simulink model "BFE_TestHarness"  (Simulink 8.6)
settings: Solver=FixedStepDiscrete  StartTime=0.0  StopTime=3  FixedStep=Ts  RelTol=1e-3
PreLoadFcn:
  | addpath('MBD_Tests')
  | 
  | load('Workspace\EnvVar.mat')
  | run('MBD_Tests\MBD_tests_init.m')
  | if exist('tl_preloadfcn','file'), tl_preloadfcn(gcs,402); end
PostLoadFcn:
  | if exist('tl_postloadfcn','file'), tl_postloadfcn(gcs,402); end
InitFcn:
  | if exist('tlds_init','file'), tlds_init(gcs); end
StartFcn:
  | if exist('tlds_start','file'), tlds_start(gcs); end
StopFcn:
  | if exist('tlds_stop','file'), tlds_stop(gcs); end
undefined symbols (not defined in the file): ddv, Ts, u2, u3, u4
libraries: tllib x11, simulink x8, LIB_TF_G_111 x2, LIB_TF_G_12_StepControl x2, LIB_TF_G_112 x1, LIB_TF_G_113 x1
(part 11 of 17)

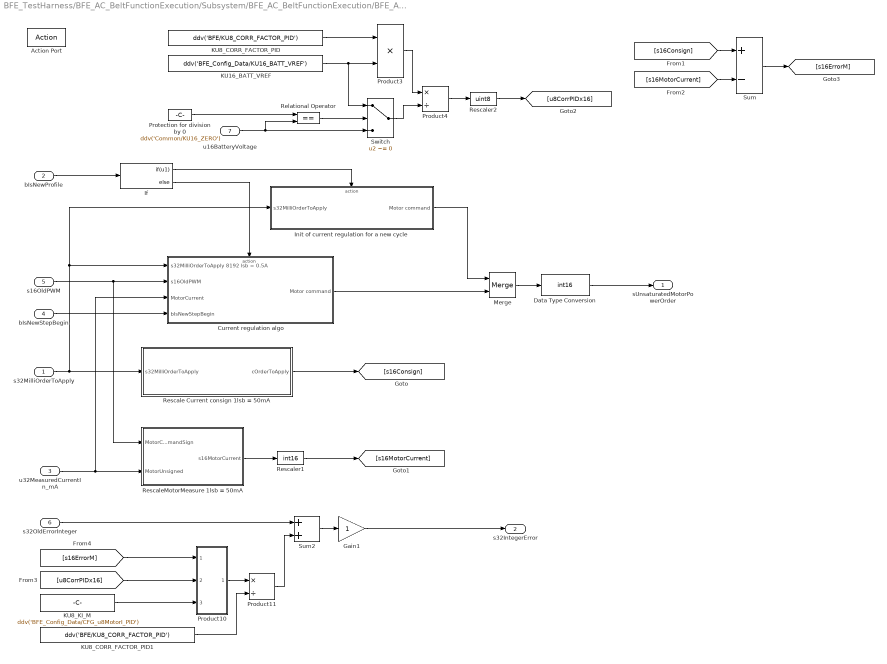
== system BFE_TestHarness/BFE_AC_BeltFunctionExecution/Subsystem/BFE_AC_BeltFunctionExecution/BFE_AC_BeltFunctionExecution/BFE_runExecuteStandardSteps/ExecuteStandardSteps/SubsystemConvertOrderToMotorPower/Current_Regulation/Standard Regulation ==
  s32MilliOrderToApply : Inport  RequirementInfo={} %GIDa_a782df3b_cd2f_48ec_84bc_b42b59744bc6
  bIsNewProfile : Inport  RequirementInfo={} %GIDa_a44577a2_8625_45c3_aeb0_51c9285d1a85  Port=2
  u32MeasuredCurrentIn_mA : Inport  RequirementInfo={} %GIDa_7c33bc16_f4d7_41a6_837e_bf2e5b8e2de6  Port=3
  bIsNewStepBegin : Inport  RequirementInfo={} %GIDa_89b8018c_31ff_454d_820a_6fb8a1af90d7  Port=4
  s16OldPWM : Inport  RequirementInfo={} %GIDa_84405069_397b_4c2d_9940_083b086742df  Port=5
  s32OldErrorInteger : Inport  RequirementInfo={} %GIDa_3b3878a2_30a5_4bd8_a4cc_60f462ef7e39  Port=6
  u16BatteryVoltage : Inport  RequirementInfo={} %GIDa_ae36fff5_70fb_4eda_b8dc_2f0f1fd7ad12  Port=7
  Action Port : ActionPort  RequirementInfo={} %GIDa_eb4ea71c_0e34_4a3e_b607_23ed5579d26c  ActionType=then
  Current regulation algo : Subsystem  TreatAsAtomicUnit=on
  Data Type Conversion : DataTypeConversion  RequirementInfo={} %GIDa_77bacd59_8a03_4be2_81ef_2d2f22f87e72  OutDataTypeStr=int16  mask(TL_Rescaler){data={'date',735951.66854917828}}
      settings: DeleteFcn=if exist('delete_tlblock','file')==2,delete_tlblock(gcbh);end  NameChangeFcn=if exist('rename_tlblock','file')==2,rename_tlblock(gcbh);end  OpenFcn=if exist('tl_open_blockdlg','file')==2,tl_open_blockdlg(gcbh);else,open_system(gcbh,'parameter');end
      mask Help: eval(['if exist(''tl_online_help'',''file'') == 2, tl_online_help(''Topic'',''TL_Rescaler''),else, web([''jar:file:///'',matlabroot,''/help/toolbox/simulink/help.jar!/slref/' lower(get_param(gcbh,'Blocktype')) '.html''], ''-helpbrowser''),end'])
      mask Display: plot([-0.05, 1.05, NaN, -0.05, 1.05],[.01, .01, NaN, .99, .99])
  Gain1 : Gain  RequirementInfo={} %GIDa_240eae8e_68ae_46cb_b8de_0b9900bc89c0  OutDataTypeStr=int32  mask(TL_Gain){data={'output',{'type','Int32'},'date',735951.66854881949}}
      settings: CopyFcn=if exist('tl_reset_reviewflag','file')==2,tl_reset_reviewflag(gcbh);end  DeleteFcn=if exist('delete_tlblock','file')==2,delete_tlblock(gcbh);end  NameChangeFcn=if exist('rename_tlblock','file')==2,rename_tlblock(gcbh);end  OpenFcn=if exist('tl_open_blockdlg','file')==2,tl_open_blockdlg(gcbh);else,open_system(gcbh,'parameter');end
      mask Help: eval(['if exist(''tl_online_help'',''file'') == 2, tl_online_help(''Topic'',''TL_Gain''),else, web([''jar:file:///'',matlabroot,''/help/toolbox/simulink/help.jar!/slref/' lower(get_param(gcbh,'Blocktype')) '.html''], ''-helpbrowser''),end'])
      mask Display: plot([0, .9, 0],[.05, .5, .95])
  If : If  IfExpression=u1
  Init of current regulation for a new cycle : Subsystem  TreatAsAtomicUnit=on
  KU16_BATT_VREF : Constant  RequirementInfo={} %GIDa_2fbae1ab_a28b_4d2e_975d_0f9f269946ee  Value=ddv('BFE_Config_Data/KU16_BATT_VREF')  OutDataTypeStr=uint16  mask(TL_Constant){data={'output',{'variable','BFE_Config_Data/KU16_BATT_VREF'},'date',735951.66854578699}}
      settings: CopyFcn=if exist('tl_reset_reviewflag','file')==2,tl_reset_reviewflag(gcbh);end  DeleteFcn=if exist('delete_tlblock','file')==2,delete_tlblock(gcbh);end  NameChangeFcn=if exist('rename_tlblock','file')==2,rename_tlblock(gcbh);end  OpenFcn=if exist('tl_open_blockdlg','file')==2,tl_open_blockdlg(gcbh);else,open_system(gcbh,'parameter');end
      mask Help: eval(['if exist(''tl_online_help'',''file'') == 2, tl_online_help(''Topic'',''TL_Constant''),else, web([''jar:file:///'',matlabroot,''/help/toolbox/simulink/help.jar!/slref/' lower(get_param(gcbh,'Blocktype')) '.html''], ''-helpbrowser''),end'])
      mask Display: plot([-0.05, 1.05, NaN, -0.05, 1.05],[.01, .01, NaN, .99, .99])
  KU8_CORR_FACTOR_PID : Constant  RequirementInfo={} %GIDa_78255bf5_403f_48d2_a530_3c6e07dfbf1a  Value=ddv('BFE/KU8_CORR_FACTOR_PID')  OutDataTypeStr=uint8  mask(TL_Constant){data={'output',{'variable','BFE/KU8_CORR_FACTOR_PID'},'date',735951.66854541667}}
      settings: CopyFcn=if exist('tl_reset_reviewflag','file')==2,tl_reset_reviewflag(gcbh);end  DeleteFcn=if exist('delete_tlblock','file')==2,delete_tlblock(gcbh);end  NameChangeFcn=if exist('rename_tlblock','file')==2,rename_tlblock(gcbh);end  OpenFcn=if exist('tl_open_blockdlg','file')==2,tl_open_blockdlg(gcbh);else,open_system(gcbh,'parameter');end
      mask Help: eval(['if exist(''tl_online_help'',''file'') == 2, tl_online_help(''Topic'',''TL_Constant''),else, web([''jar:file:///'',matlabroot,''/help/toolbox/simulink/help.jar!/slref/' lower(get_param(gcbh,'Blocktype')) '.html''], ''-helpbrowser''),end'])
      mask Display: plot([-0.05, 1.05, NaN, -0.05, 1.05],[.01, .01, NaN, .99, .99])
  KU8_CORR_FACTOR_PID1 : Constant  RequirementInfo={} %GIDa_3c653f60_82b8_4086_9e8c_c5b737d3d0e8  Value=ddv('BFE/KU8_CORR_FACTOR_PID')  OutDataTypeStr=uint8  mask(TL_Constant){data={'output',{'variable','BFE/KU8_CORR_FACTOR_PID'},'date',735951.66854503471}}
      settings: CopyFcn=if exist('tl_reset_reviewflag','file')==2,tl_reset_reviewflag(gcbh);end  DeleteFcn=if exist('delete_tlblock','file')==2,delete_tlblock(gcbh);end  NameChangeFcn=if exist('rename_tlblock','file')==2,rename_tlblock(gcbh);end  OpenFcn=if exist('tl_open_blockdlg','file')==2,tl_open_blockdlg(gcbh);else,open_system(gcbh,'parameter');end
      mask Help: eval(['if exist(''tl_online_help'',''file'') == 2, tl_online_help(''Topic'',''TL_Constant''),else, web([''jar:file:///'',matlabroot,''/help/toolbox/simulink/help.jar!/slref/' lower(get_param(gcbh,'Blocktype')) '.html''], ''-helpbrowser''),end'])
      mask Display: plot([-0.05, 1.05, NaN, -0.05, 1.05],[.01, .01, NaN, .99, .99])
  KU8_KI_M : Constant  RequirementInfo={} %GIDa_2b7a27a1_c83e_482d_9a98_41e7f4309a04  Value=ddv('BFE_Config_Data/CFG_u8MotorI_PID')  OutDataTypeStr=uint8  mask(TL_Constant){data={'output',{'variable','BFE_Config_Data/CFG_u8MotorI_PID'},'date',735951.66854465276}}
      settings: CopyFcn=if exist('tl_reset_reviewflag','file')==2,tl_reset_reviewflag(gcbh);end  DeleteFcn=if exist('delete_tlblock','file')==2,delete_tlblock(gcbh);end  NameChangeFcn=if exist('rename_tlblock','file')==2,rename_tlblock(gcbh);end  OpenFcn=if exist('tl_open_blockdlg','file')==2,tl_open_blockdlg(gcbh);else,open_system(gcbh,'parameter');end
      mask Help: eval(['if exist(''tl_online_help'',''file'') == 2, tl_online_help(''Topic'',''TL_Constant''),else, web([''jar:file:///'',matlabroot,''/help/toolbox/simulink/help.jar!/slref/' lower(get_param(gcbh,'Blocktype')) '.html''], ''-helpbrowser''),end'])
      mask Display: plot([-0.05, 1.05, NaN, -0.05, 1.05],[.01, .01, NaN, .99, .99])
  Merge : Merge  InitialOutput=0  mask(TL_Merge){data={'date',735951.6685442708}}
      settings: CopyFcn=if exist('tl_reset_reviewflag','file')==2,tl_reset_reviewflag(gcbh);end  DeleteFcn=if exist('delete_tlblock','file')==2,delete_tlblock(gcbh);end  NameChangeFcn=if exist('rename_tlblock','file')==2,rename_tlblock(gcbh);end  OpenFcn=if exist('tl_open_blockdlg','file')==2,tl_open_blockdlg(gcbh);else,open_system(gcbh,'parameter');end
      mask Help: eval(['if exist(''tl_online_help'',''file'') == 2, tl_online_help(''Topic'',''TL_Merge''),else, web([''jar:file:///'',matlabroot,''/help/toolbox/simulink/help.jar!/slref/' lower(get_param(gcbh,'Blocktype')) '.html''], ''-helpbrowser''),end'])
      mask Display: plot([-0.05, 1.05, NaN, -0.05, 1.05],[.01, .01, NaN, .99, .99])
  Product10 : Subsystem  RequirementInfo={} %GIDa_f767c257_68db_48eb_9874_98d302407301
      mask Display: plot([4 10 NaN 4 10 ],[82 88 NaN 88 82 ]);plot([4 10 NaN 4 10 ],[47 53 NaN 53 47 ]);plot([4 10 NaN 4 10 ],[12 18 NaN 18 12 ]);
  Product11 : Product  RequirementInfo={} %GIDa_05da5e16_588f_40e9_b405_55adb34adf78  Inputs=*/  RndMeth=Zero  mask(TL_Product){data={'output',{'type','Int32'},'date',735951.66854312504}}
      settings: CopyFcn=if exist('tl_reset_reviewflag','file')==2,tl_reset_reviewflag(gcbh);end  DeleteFcn=if exist('delete_tlblock','file')==2,delete_tlblock(gcbh);end  NameChangeFcn=if exist('rename_tlblock','file')==2,rename_tlblock(gcbh);end  OpenFcn=if exist('tl_open_blockdlg','file')==2,tl_open_blockdlg(gcbh);else,open_system(gcbh,'parameter');end
      mask Help: eval(['if exist(''tl_online_help'',''file'') == 2, tl_online_help(''Topic'',''TL_Product''),else, web([''jar:file:///'',matlabroot,''/help/toolbox/simulink/help.jar!/slref/' lower(get_param(gcbh,'Blocktype')) '.html''], ''-helpbrowser''),end'])
      mask Display: plot([-0.05, 1.05, NaN, -0.05, 1.05],[.01, .01, NaN, .99, .99])
  Product3 : Product  RequirementInfo={} %GIDa_5e53fb6f_ceab_4fe0_9d47_7ec7af3cf549  Inputs=**  RndMeth=Zero  mask(TL_Product){data={'output',{'type','UInt32'},'date',735951.66854276625}}
      settings: CopyFcn=if exist('tl_reset_reviewflag','file')==2,tl_reset_reviewflag(gcbh);end  DeleteFcn=if exist('delete_tlblock','file')==2,delete_tlblock(gcbh);end  NameChangeFcn=if exist('rename_tlblock','file')==2,rename_tlblock(gcbh);end  OpenFcn=if exist('tl_open_blockdlg','file')==2,tl_open_blockdlg(gcbh);else,open_system(gcbh,'parameter');end
      mask Help: eval(['if exist(''tl_online_help'',''file'') == 2, tl_online_help(''Topic'',''TL_Product''),else, web([''jar:file:///'',matlabroot,''/help/toolbox/simulink/help.jar!/slref/' lower(get_param(gcbh,'Blocktype')) '.html''], ''-helpbrowser''),end'])
      mask Display: plot([-0.05, 1.05, NaN, -0.05, 1.05],[.01, .01, NaN, .99, .99])
  Product4 : Product  RequirementInfo={} %GIDa_70232b70_1706_4488_b9fd_672dede75738  Inputs=*/  RndMeth=Zero  mask(TL_Product){data={'output',{'type','UInt32'},'exceptionhandling',0,'date',735951.66854238429}}
      settings: CopyFcn=if exist('tl_reset_reviewflag','file')==2,tl_reset_reviewflag(gcbh);end  DeleteFcn=if exist('delete_tlblock','file')==2,delete_tlblock(gcbh);end  NameChangeFcn=if exist('rename_tlblock','file')==2,rename_tlblock(gcbh);end  OpenFcn=if exist('tl_open_blockdlg','file')==2,tl_open_blockdlg(gcbh);else,open_system(gcbh,'parameter');end
      mask Help: eval(['if exist(''tl_online_help'',''file'') == 2, tl_online_help(''Topic'',''TL_Product''),else, web([''jar:file:///'',matlabroot,''/help/toolbox/simulink/help.jar!/slref/' lower(get_param(gcbh,'Blocktype')) '.html''], ''-helpbrowser''),end'])
      mask Display: plot([-0.05, 1.05, NaN, -0.05, 1.05],[.01, .01, NaN, .99, .99])
  Protection for division by 0 : Constant  Value=ddv('Common/KU16_ZERO')  mask(TL_Constant){data={'output',{'variable','Common/KU16_ZERO'},'date',735951.66854201385}}
      settings: CopyFcn=if exist('tl_reset_reviewflag','file')==2,tl_reset_reviewflag(gcbh);end  DeleteFcn=if exist('delete_tlblock','file')==2,delete_tlblock(gcbh);end  NameChangeFcn=if exist('rename_tlblock','file')==2,rename_tlblock(gcbh);end  OpenFcn=if exist('tl_open_blockdlg','file')==2,tl_open_blockdlg(gcbh);else,open_system(gcbh,'parameter');end
      mask Help: eval(['if exist(''tl_online_help'',''file'') == 2, tl_online_help(''Topic'',''TL_Constant''),else, web([''jar:file:///'',matlabroot,''/help/toolbox/simulink/help.jar!/slref/' lower(get_param(gcbh,'Blocktype')) '.html''], ''-helpbrowser''),end'])
      mask Display: plot([-0.05, 1.05, NaN, -0.05, 1.05],[.01, .01, NaN, .99, .99])
  Relational Operator : RelationalOperator  Operator===  OutDataTypeStr=boolean  mask(TL_RelationalOperator){data={'date',735951.66854165506}}
      settings: DeleteFcn=if exist('delete_tlblock','file')==2,delete_tlblock(gcbh);end  NameChangeFcn=if exist('rename_tlblock','file')==2,rename_tlblock(gcbh);end  OpenFcn=if exist('tl_open_blockdlg','file')==2,tl_open_blockdlg(gcbh);else,open_system(gcbh,'parameter');end
      mask Help: eval(['if exist(''tl_online_help'',''file'') == 2, tl_online_help(''Topic'',''TL_RelationalOperator''),else, web([''jar:file:///'',matlabroot,''/help/toolbox/simulink/help.jar!/slref/' lower(get_param(gcbh,'Blocktype')) '.html''], ''-helpbrowser''),end'])
      mask Display: plot([-0.05, 1.05, NaN, -0.05, 1.05],[.01, .01, NaN, .99, .99])
  Rescale Current consign 1lsb = 50mA : Subsystem  RequirementInfo={} %GIDa_fdff63d8_bdcf_4376_a137_337af77cbfb4
  RescaleMotorMeasure 1lsb = 50mA : Subsystem  RequirementInfo={} %GIDa_d2c6756e_dc23_445d_b4ca_0746f033342a  TreatAsAtomicUnit=on
  Rescaler1 : DataTypeConversion  RequirementInfo={} %GIDa_044cb36d_c668_4fc2_a10d_86685e254bcb  OutDataTypeStr=int16  SaturateOnIntegerOverflow=on  RndMeth=Zero  mask(TL_Rescaler){data={'output',{'name','s16MotorCurrentM_204'},'date',735951.66853535874}}
      settings: DeleteFcn=if exist('delete_tlblock','file')==2,delete_tlblock(gcbh);end  NameChangeFcn=if exist('rename_tlblock','file')==2,rename_tlblock(gcbh);end  OpenFcn=if exist('tl_open_blockdlg','file')==2,tl_open_blockdlg(gcbh);else,open_system(gcbh,'parameter');end
      mask Help: eval(['if exist(''tl_online_help'',''file'') == 2, tl_online_help(''Topic'',''TL_Rescaler''),else, web([''jar:file:///'',matlabroot,''/help/toolbox/simulink/help.jar!/slref/' lower(get_param(gcbh,'Blocktype')) '.html''], ''-helpbrowser''),end'])
      mask Display: plot([-0.05, 1.05, NaN, -0.05, 1.05],[.01, .01, NaN, .99, .99])
  Rescaler2 : DataTypeConversion  RequirementInfo={} %GIDa_26de5298_a930_4926_bcb3_9f8f9b842192  OutDataTypeStr=uint8  SaturateOnIntegerOverflow=on  RndMeth=Zero  mask(TL_Rescaler){data={'output',{'name','u8CorrPIDx16_204','type','UInt8'},'date',735951.66853504628}}
      settings: DeleteFcn=if exist('delete_tlblock','file')==2,delete_tlblock(gcbh);end  NameChangeFcn=if exist('rename_tlblock','file')==2,rename_tlblock(gcbh);end  OpenFcn=if exist('tl_open_blockdlg','file')==2,tl_open_blockdlg(gcbh);else,open_system(gcbh,'parameter');end
      mask Help: eval(['if exist(''tl_online_help'',''file'') == 2, tl_online_help(''Topic'',''TL_Rescaler''),else, web([''jar:file:///'',matlabroot,''/help/toolbox/simulink/help.jar!/slref/' lower(get_param(gcbh,'Blocktype')) '.html''], ''-helpbrowser''),end'])
      mask Display: plot([-0.05, 1.05, NaN, -0.05, 1.05],[.01, .01, NaN, .99, .99])
  Sum : Sum  RequirementInfo={} %GIDa_21aea4e4_1c5d_4da0_972e_0efc7a1f84ed  Inputs=+-  mask(TL_Sum){data={'output',{'name','s16ErrorM_204'},'date',735951.66853471065}}
      settings: CopyFcn=if exist('tl_reset_reviewflag','file')==2,tl_reset_reviewflag(gcbh);end  DeleteFcn=if exist('delete_tlblock','file')==2,delete_tlblock(gcbh);end  NameChangeFcn=if exist('rename_tlblock','file')==2,rename_tlblock(gcbh);end  OpenFcn=if exist('tl_open_blockdlg','file')==2,tl_open_blockdlg(gcbh);else,open_system(gcbh,'parameter');end
      mask Help: eval(['if exist(''tl_online_help'',''file'') == 2, tl_online_help(''Topic'',''TL_Sum''),else, web([''jar:file:///'',matlabroot,''/help/toolbox/simulink/help.jar!/slref/' lower(get_param(gcbh,'Blocktype')) '.html''], ''-helpbrowser''),end'])
      mask Display: plot([-0.05, 1.05, NaN, -0.05, 1.05],[.01, .01, NaN, .99, .99])
  Sum2 : Sum  RequirementInfo={} %GIDa_070b8bc6_ad2d_4c77_accf_3ff0a1d37eb1  mask(TL_Sum){data={'output',{'type','Int32'},'date',735951.66853435186}}
      settings: CopyFcn=if exist('tl_reset_reviewflag','file')==2,tl_reset_reviewflag(gcbh);end  DeleteFcn=if exist('delete_tlblock','file')==2,delete_tlblock(gcbh);end  NameChangeFcn=if exist('rename_tlblock','file')==2,rename_tlblock(gcbh);end  OpenFcn=if exist('tl_open_blockdlg','file')==2,tl_open_blockdlg(gcbh);else,open_system(gcbh,'parameter');end
      mask Help: eval(['if exist(''tl_online_help'',''file'') == 2, tl_online_help(''Topic'',''TL_Sum''),else, web([''jar:file:///'',matlabroot,''/help/toolbox/simulink/help.jar!/slref/' lower(get_param(gcbh,'Blocktype')) '.html''], ''-helpbrowser''),end'])
      mask Display: plot([-0.05, 1.05, NaN, -0.05, 1.05],[.01, .01, NaN, .99, .99])
  Switch : Switch  Criteria=u2 ~= 0  mask(TL_Switch){data={'output',{'name','u16BattVoltFiltered_$B','type','UInt16'},'date',735951.66853395838}}
      settings: CopyFcn=if exist('tl_reset_reviewflag','file')==2,tl_reset_reviewflag(gcbh);end  DeleteFcn=if exist('delete_tlblock','file')==2,delete_tlblock(gcbh);end  NameChangeFcn=if exist('rename_tlblock','file')==2,rename_tlblock(gcbh);end  OpenFcn=if exist('tl_open_blockdlg','file')==2,tl_open_blockdlg(gcbh);else,open_system(gcbh,'parameter');end
      mask Help: eval(['if exist(''tl_online_help'',''file'') == 2, tl_online_help(''Topic'',''TL_Switch''),else, web([''jar:file:///'',matlabroot,''/help/toolbox/simulink/help.jar!/slref/' lower(get_param(gcbh,'Blocktype')) '.html''], ''-helpbrowser''),end'])
      mask Display: plot([-0.05, 1.05, NaN, -0.05, 1.05],[.01, .01, NaN, .99, .99])
  sUnsaturatedMotorPowerOrder : Outport  RequirementInfo={} %GIDa_b57bec31_362d_4b2e_a7be_1b9028a374c3  InitialOutput=0
  s32IntegerError : Outport  RequirementInfo={} %GIDa_4885f9c4_4183_439d_8537_24cbc622a798  Port=2  InitialOutput=0
  wires:
  s32MilliOrderToApply/1 -> Rescale Current consign 1lsb = 50mA/1(s32MilliOrderToApply), Current regulation algo/1(s32MilliOrderToApply 8192 lsb = 0.5A), Init of current regulation for a new cycle/1(s32MilliOrderToApply)
  u32MeasuredCurrentIn_mA/1 -> RescaleMotorMeasure 1lsb = 50mA/2(MotorUnsigned), Current regulation algo/3(MotorCurrent)
  Product11/1 -> Sum2/2
  KU8_CORR_FACTOR_PID1/1 -> Product11/2
  Product10/1(Out_1) -> Product11/1
  KU8_KI_M/1 -> Product10/3(In_3)
  [u8CorrPIDx16] -> Product10/2(In_2)
  Sum2/1 -> Gain1/1
  Gain1/1 -> s32IntegerError/1
  s32OldErrorInteger/1 -> Sum2/1
  RescaleMotorMeasure 1lsb = 50mA/1(s16MotorCurrent) -> Rescaler1/1
  Rescaler1/1 -> [s16MotorCurrent]
  [s16Consign] -> Sum/1
  [s16MotorCurrent] -> Sum/2
  Sum/1 -> [s16ErrorM]
  KU8_CORR_FACTOR_PID/1 -> Product3/1
  KU16_BATT_VREF/1 -> Product3/2, Switch/1
  Product3/1 -> Product4/1
  Product4/1 -> Rescaler2/1
  Rescaler2/1 -> [u8CorrPIDx16]
  [s16ErrorM] -> Product10/1(In_1)
  Protection for division by 0/1 -> Relational Operator/1
  Relational Operator/1 -> Switch/2
  u16BatteryVoltage/1 -> Relational Operator/2, Switch/3
  Switch/1 -> Product4/2
  If/1 -> Init of current regulation for a new cycle/Action
  bIsNewProfile/1 -> If/1
  If/2 -> Current regulation algo/Action
  Init of current regulation for a new cycle/1(Motor command) -> Merge/1
  Current regulation algo/1(Motor command) -> Merge/2
  Merge/1 -> Data Type Conversion/1
  Rescale Current consign 1lsb = 50mA/1(cOrderToApply) -> [s16Consign]
  Data Type Conversion/1 -> sUnsaturatedMotorPowerOrder/1
  s16OldPWM/1 -> RescaleMotorMeasure 1lsb = 50mA/1(MotorCommandSign), Current regulation algo/2(s16OldPWM)
  bIsNewStepBegin/1 -> Current regulation algo/4(bIsNewStepBegin)

== system BFE_TestHarness/BFE_AC_BeltFunctionExecution/Subsystem/BFE_AC_BeltFunctionExecution/BFE_AC_BeltFunctionExecution/BFE_runExecuteStandardSteps/ExecuteStandardSteps/SubsystemConvertOrderToMotorPower/MotorVoltage_Regulation/Battery voltage rescaling ==
  note: Add a default battery value if ADC value is not available ?
  note: This operation will overflow if Vbatt > 524 V !
      | Which seems out of range for our design. No problem here
  note: Convert from 1 LSB / mV to 0.25 LSB / V
  note: Rescale battery voltage to match order value unit and resolution
  usBatteryVoltage : Inport
  Constant : Constant  Value=ddv('BFE/KUC_NEUTRAL_WEIGHT')  mask(TL_Constant){data={'output',{'variable','BFE/KUC_NEUTRAL_WEIGHT'},'date',737167.44609568291}}
      settings: CopyFcn=if exist('tl_reset_reviewflag') == 2, tl_reset_reviewflag(gcbh); end  DeleteFcn=if exist('delete_tlblock','file')==2,delete_tlblock(gcbh);end  NameChangeFcn=if exist('rename_tlblock','file')==2,rename_tlblock(gcbh);end  OpenFcn=if exist('tl_open_blockdlg','file')==2,tl_open_blockdlg(gcbh);else,open_system(gcbh,'parameter');end
      mask Help: eval(['if exist(''tl_online_help'',''file'') == 2, tl_online_help(''Topic'',''TL_Constant''),else, web([''jar:file:///'',matlabroot,''/help/toolbox/simulink/help.jar!/slref/' lower(get_param(gcbh,'Blocktype')) '.html''], ''-helpbrowser''),end'])
      mask Display: plot([-0.1, 1.05, NaN, -0.1, 1.05],[.01, .01, NaN, .99, .99]);
  Constant1 : Constant  Value=ddv('BFE/KUS_MOTOR_VOLTAGE_ORDER_RES')  mask(TL_Constant){data={'output',{'variable','BFE/KUS_MOTOR_VOLTAGE_ORDER_RES'},'date',737167.44629472226}}
      settings: CopyFcn=if exist('tl_reset_reviewflag') == 2, tl_reset_reviewflag(gcbh); end  DeleteFcn=if exist('delete_tlblock','file')==2,delete_tlblock(gcbh);end  NameChangeFcn=if exist('rename_tlblock','file')==2,rename_tlblock(gcbh);end  OpenFcn=if exist('tl_open_blockdlg','file')==2,tl_open_blockdlg(gcbh);else,open_system(gcbh,'parameter');end
      mask Help: eval(['if exist(''tl_online_help'',''file'') == 2, tl_online_help(''Topic'',''TL_Constant''),else, web([''jar:file:///'',matlabroot,''/help/toolbox/simulink/help.jar!/slref/' lower(get_param(gcbh,'Blocktype')) '.html''], ''-helpbrowser''),end'])
      mask Display: plot([-0.1, 1.05, NaN, -0.1, 1.05],[.01, .01, NaN, .99, .99]);
  Constant2 : Constant  Value=ddv('BFE/KU8_NO_POWER_ADAPT')  mask(TL_Constant){data={'output',{'variable','BFE/KU8_NO_POWER_ADAPT'},'date',737167.44660471065}}
      settings: CopyFcn=if exist('tl_reset_reviewflag') == 2, tl_reset_reviewflag(gcbh); end  DeleteFcn=if exist('delete_tlblock','file')==2,delete_tlblock(gcbh);end  NameChangeFcn=if exist('rename_tlblock','file')==2,rename_tlblock(gcbh);end  OpenFcn=if exist('tl_open_blockdlg','file')==2,tl_open_blockdlg(gcbh);else,open_system(gcbh,'parameter');end
      mask Help: eval(['if exist(''tl_online_help'',''file'') == 2, tl_online_help(''Topic'',''TL_Constant''),else, web([''jar:file:///'',matlabroot,''/help/toolbox/simulink/help.jar!/slref/' lower(get_param(gcbh,'Blocktype')) '.html''], ''-helpbrowser''),end'])
      mask Display: plot([-0.1, 1.05, NaN, -0.1, 1.05],[.01, .01, NaN, .99, .99]);
  Product : Product  Inputs=**  RndMeth=Zero  mask(TL_Product){data={'output',{'type','UInt32'},'date',737167.44390218752}}
      settings: CopyFcn=if exist('tl_reset_reviewflag') == 2, tl_reset_reviewflag(gcbh); end  DeleteFcn=if exist('delete_tlblock','file')==2,delete_tlblock(gcbh);end  NameChangeFcn=if exist('rename_tlblock','file')==2,rename_tlblock(gcbh);end  OpenFcn=if exist('tl_open_blockdlg','file')==2,tl_open_blockdlg(gcbh);else,open_system(gcbh,'parameter');end
      mask Help: eval(['if exist(''tl_online_help'',''file'') == 2, tl_online_help(''Topic'',''TL_Product''),else, web([''jar:file:///'',matlabroot,''/help/toolbox/simulink/help.jar!/slref/' lower(get_param(gcbh,'Blocktype')) '.html''], ''-helpbrowser''),end'])
      mask Display: plot([-0.1, 1.05, NaN, -0.1, 1.05],[.01, .01, NaN, .99, .99]);
  Product1 : Product  Inputs=**  RndMeth=Zero  mask(TL_Product){data={'output',{'type','UInt32'},'date',737167.44380883104}}
      settings: CopyFcn=if exist('tl_reset_reviewflag') == 2, tl_reset_reviewflag(gcbh); end  DeleteFcn=if exist('delete_tlblock','file')==2,delete_tlblock(gcbh);end  NameChangeFcn=if exist('rename_tlblock','file')==2,rename_tlblock(gcbh);end  OpenFcn=if exist('tl_open_blockdlg','file')==2,tl_open_blockdlg(gcbh);else,open_system(gcbh,'parameter');end
      mask Help: eval(['if exist(''tl_online_help'',''file'') == 2, tl_online_help(''Topic'',''TL_Product''),else, web([''jar:file:///'',matlabroot,''/help/toolbox/simulink/help.jar!/slref/' lower(get_param(gcbh,'Blocktype')) '.html''], ''-helpbrowser''),end'])
      mask Display: plot([-0.1, 1.05, NaN, -0.1, 1.05],[.01, .01, NaN, .99, .99]);
  usBattVoltageScaled : Product  Inputs=*/  RndMeth=Zero  mask(TL_Product){data={'output',{'type','UInt32'},'date',737167.55372688663}}
      settings: CopyFcn=if exist('tl_reset_reviewflag') == 2, tl_reset_reviewflag(gcbh); end  DeleteFcn=if exist('delete_tlblock','file')==2,delete_tlblock(gcbh);end  NameChangeFcn=if exist('rename_tlblock','file')==2,rename_tlblock(gcbh);end  OpenFcn=if exist('tl_open_blockdlg','file')==2,tl_open_blockdlg(gcbh);else,open_system(gcbh,'parameter');end
      mask Help: eval(['if exist(''tl_online_help'',''file'') == 2, tl_online_help(''Topic'',''TL_Product''),else, web([''jar:file:///'',matlabroot,''/help/toolbox/simulink/help.jar!/slref/' lower(get_param(gcbh,'Blocktype')) '.html''], ''-helpbrowser''),end'])
      mask Display: plot([-0.1, 1.05, NaN, -0.1, 1.05],[.01, .01, NaN, .99, .99]);
  usBatteryVoltageScaled : Outport
  wires:
  usBatteryVoltage/1 -> Product/1
  Constant2/1 -> Product/2
  Product/1 -> Product1/1
  Constant/1 -> Product1/2
  Product1/1 -> usBattVoltageScaled/1
  Constant1/1 -> usBattVoltageScaled/2
  usBattVoltageScaled/1 -> usBatteryVoltageScaled/1

== system BFE_TestHarness/BFE_AC_BeltFunctionExecution/Subsystem/BFE_AC_BeltFunctionExecution/BFE_AC_BeltFunctionExecution/BFE_runExecuteStandardSteps/ExecuteStandardSteps/SubsystemConvertOrderToMotorPower/MotorVoltage_Regulation/Consign < Battery voltage => Compute PWM ==
  lOrderToApply : Inport  RequirementInfo={} %GIDa_96bc9362_0989_4bcb_aca1_2d11e1b24c87
  usBatteryVoltage : Inport  RequirementInfo={} %GIDa_c11bb75d_867f_42d9_96c2_cf6c5b0350ea  Port=2
  Action Port : ActionPort  ActionType=else
  Arrondi 1/2 lsb : Constant  Value=ddv('BFE/ExecuteStdSteps_Rescaling/KU16_VOLT_RSC_NUM2')  mask(TL_Constant){data={'output',{'variable','BFE/ExecuteStdSteps_Rescaling/KU16_VOLT_RSC_NUM2'},'date',735951.66852520837}}
      settings: CopyFcn=if exist('tl_reset_reviewflag','file')==2,tl_reset_reviewflag(gcbh);end  DeleteFcn=if exist('delete_tlblock','file')==2,delete_tlblock(gcbh);end  NameChangeFcn=if exist('rename_tlblock','file')==2,rename_tlblock(gcbh);end  OpenFcn=if exist('tl_open_blockdlg','file')==2,tl_open_blockdlg(gcbh);else,open_system(gcbh,'parameter');end
      mask Help: eval(['if exist(''tl_online_help'',''file'') == 2, tl_online_help(''Topic'',''TL_Constant''),else, web([''jar:file:///'',matlabroot,''/help/toolbox/simulink/help.jar!/slref/' lower(get_param(gcbh,'Blocktype')) '.html''], ''-helpbrowser''),end'])
      mask Display: plot([-0.05, 1.05, NaN, -0.05, 1.05],[.01, .01, NaN, .99, .99])
  Default value for Battery Voltage : Constant  Value=ddv('BFE_Config_Data/KU16_BATT_VREF')  mask(TL_Constant){data={'output',{'variable','BFE_Config_Data/KU16_BATT_VREF'},'date',735951.66852482641}}
      settings: CopyFcn=if exist('tl_reset_reviewflag','file')==2,tl_reset_reviewflag(gcbh);end  DeleteFcn=if exist('delete_tlblock','file')==2,delete_tlblock(gcbh);end  NameChangeFcn=if exist('rename_tlblock','file')==2,rename_tlblock(gcbh);end  OpenFcn=if exist('tl_open_blockdlg','file')==2,tl_open_blockdlg(gcbh);else,open_system(gcbh,'parameter');end
      mask Help: eval(['if exist(''tl_online_help'',''file'') == 2, tl_online_help(''Topic'',''TL_Constant''),else, web([''jar:file:///'',matlabroot,''/help/toolbox/simulink/help.jar!/slref/' lower(get_param(gcbh,'Blocktype')) '.html''], ''-helpbrowser''),end'])
      mask Display: plot([-0.05, 1.05, NaN, -0.05, 1.05],[.01, .01, NaN, .99, .99])
  Divider to rescale output : Constant  Value=ddv('BFE/ExecuteStdSteps_Rescaling/KU16_VOLT_RSC_DEN')  mask(TL_Constant){data={'output',{'variable','BFE/ExecuteStdSteps_Rescaling/KU16_VOLT_RSC_DEN'},'date',735951.66852444445}}
      settings: CopyFcn=if exist('tl_reset_reviewflag','file')==2,tl_reset_reviewflag(gcbh);end  DeleteFcn=if exist('delete_tlblock','file')==2,delete_tlblock(gcbh);end  NameChangeFcn=if exist('rename_tlblock','file')==2,rename_tlblock(gcbh);end  OpenFcn=if exist('tl_open_blockdlg','file')==2,tl_open_blockdlg(gcbh);else,open_system(gcbh,'parameter');end
      mask Help: eval(['if exist(''tl_online_help'',''file'') == 2, tl_online_help(''Topic'',''TL_Constant''),else, web([''jar:file:///'',matlabroot,''/help/toolbox/simulink/help.jar!/slref/' lower(get_param(gcbh,'Blocktype')) '.html''], ''-helpbrowser''),end'])
      mask Display: plot([-0.05, 1.05, NaN, -0.05, 1.05],[.01, .01, NaN, .99, .99])
  Product : Product  Inputs=**  RndMeth=Zero  mask(TL_Product){data={'output',{'type','Int32'},'date',735951.66852406249}}
      settings: CopyFcn=if exist('tl_reset_reviewflag','file')==2,tl_reset_reviewflag(gcbh);end  DeleteFcn=if exist('delete_tlblock','file')==2,delete_tlblock(gcbh);end  NameChangeFcn=if exist('rename_tlblock','file')==2,rename_tlblock(gcbh);end  OpenFcn=if exist('tl_open_blockdlg','file')==2,tl_open_blockdlg(gcbh);else,open_system(gcbh,'parameter');end
      mask Help: eval(['if exist(''tl_online_help'',''file'') == 2, tl_online_help(''Topic'',''TL_Product''),else, web([''jar:file:///'',matlabroot,''/help/toolbox/simulink/help.jar!/slref/' lower(get_param(gcbh,'Blocktype')) '.html''], ''-helpbrowser''),end'])
      mask Display: plot([-0.05, 1.05, NaN, -0.05, 1.05],[.01, .01, NaN, .99, .99])
  Product1 : Product  Inputs=*/  RndMeth=Zero  mask(TL_Product){data={'output',{'name','s32TempVoltageData','type','Int32'},'date',735951.6685237037}}
      settings: CopyFcn=if exist('tl_reset_reviewflag','file')==2,tl_reset_reviewflag(gcbh);end  DeleteFcn=if exist('delete_tlblock','file')==2,delete_tlblock(gcbh);end  NameChangeFcn=if exist('rename_tlblock','file')==2,rename_tlblock(gcbh);end  OpenFcn=if exist('tl_open_blockdlg','file')==2,tl_open_blockdlg(gcbh);else,open_system(gcbh,'parameter');end
      mask Help: eval(['if exist(''tl_online_help'',''file'') == 2, tl_online_help(''Topic'',''TL_Product''),else, web([''jar:file:///'',matlabroot,''/help/toolbox/simulink/help.jar!/slref/' lower(get_param(gcbh,'Blocktype')) '.html''], ''-helpbrowser''),end'])
      mask Display: plot([-0.05, 1.05, NaN, -0.05, 1.05],[.01, .01, NaN, .99, .99])
  Product2 : Product  Inputs=**  RndMeth=Zero  mask(TL_Product){data={'output',{'type','Int32'},'date',735951.66852333338}}
      settings: CopyFcn=if exist('tl_reset_reviewflag','file')==2,tl_reset_reviewflag(gcbh);end  DeleteFcn=if exist('delete_tlblock','file')==2,delete_tlblock(gcbh);end  NameChangeFcn=if exist('rename_tlblock','file')==2,rename_tlblock(gcbh);end  OpenFcn=if exist('tl_open_blockdlg','file')==2,tl_open_blockdlg(gcbh);else,open_system(gcbh,'parameter');end
      mask Help: eval(['if exist(''tl_online_help'',''file'') == 2, tl_online_help(''Topic'',''TL_Product''),else, web([''jar:file:///'',matlabroot,''/help/toolbox/simulink/help.jar!/slref/' lower(get_param(gcbh,'Blocktype')) '.html''], ''-helpbrowser''),end'])
      mask Display: plot([-0.05, 1.05, NaN, -0.05, 1.05],[.01, .01, NaN, .99, .99])
  Product3 : Product  Inputs=**  RndMeth=Zero  mask(TL_Product){data={'output',{'type','Int32'},'date',735951.66852296295}}
      settings: CopyFcn=if exist('tl_reset_reviewflag','file')==2,tl_reset_reviewflag(gcbh);end  DeleteFcn=if exist('delete_tlblock','file')==2,delete_tlblock(gcbh);end  NameChangeFcn=if exist('rename_tlblock','file')==2,rename_tlblock(gcbh);end  OpenFcn=if exist('tl_open_blockdlg','file')==2,tl_open_blockdlg(gcbh);else,open_system(gcbh,'parameter');end
      mask Help: eval(['if exist(''tl_online_help'',''file'') == 2, tl_online_help(''Topic'',''TL_Product''),else, web([''jar:file:///'',matlabroot,''/help/toolbox/simulink/help.jar!/slref/' lower(get_param(gcbh,'Blocktype')) '.html''], ''-helpbrowser''),end'])
      mask Display: plot([-0.05, 1.05, NaN, -0.05, 1.05],[.01, .01, NaN, .99, .99])
  Product4 : Product  Inputs=*/  RndMeth=Zero  mask(TL_Product){data={'output',{'name','s32VoltConsignBeforeSat','type','Int32'},'exceptionhandling',0,'date',735951.66852259263}}
      settings: CopyFcn=if exist('tl_reset_reviewflag','file')==2,tl_reset_reviewflag(gcbh);end  DeleteFcn=if exist('delete_tlblock','file')==2,delete_tlblock(gcbh);end  NameChangeFcn=if exist('rename_tlblock','file')==2,rename_tlblock(gcbh);end  OpenFcn=if exist('tl_open_blockdlg','file')==2,tl_open_blockdlg(gcbh);else,open_system(gcbh,'parameter');end
      mask Help: eval(['if exist(''tl_online_help'',''file'') == 2, tl_online_help(''Topic'',''TL_Product''),else, web([''jar:file:///'',matlabroot,''/help/toolbox/simulink/help.jar!/slref/' lower(get_param(gcbh,'Blocktype')) '.html''], ''-helpbrowser''),end'])
      mask Display: plot([-0.05, 1.05, NaN, -0.05, 1.05],[.01, .01, NaN, .99, .99])
  Protection for division by 0 : Constant  Value=ddv('Common/KU16_ZERO')  mask(TL_Constant){data={'output',{'variable','Common/KU16_ZERO'},'date',735951.66852223384}}
      settings: CopyFcn=if exist('tl_reset_reviewflag','file')==2,tl_reset_reviewflag(gcbh);end  DeleteFcn=if exist('delete_tlblock','file')==2,delete_tlblock(gcbh);end  NameChangeFcn=if exist('rename_tlblock','file')==2,rename_tlblock(gcbh);end  OpenFcn=if exist('tl_open_blockdlg','file')==2,tl_open_blockdlg(gcbh);else,open_system(gcbh,'parameter');end
      mask Help: eval(['if exist(''tl_online_help'',''file'') == 2, tl_online_help(''Topic'',''TL_Constant''),else, web([''jar:file:///'',matlabroot,''/help/toolbox/simulink/help.jar!/slref/' lower(get_param(gcbh,'Blocktype')) '.html''], ''-helpbrowser''),end'])
      mask Display: plot([-0.05, 1.05, NaN, -0.05, 1.05],[.01, .01, NaN, .99, .99])
  Relational Operator : RelationalOperator  Operator===  OutDataTypeStr=boolean  mask(TL_RelationalOperator){data={'date',735951.66852186341}}
      settings: DeleteFcn=if exist('delete_tlblock','file')==2,delete_tlblock(gcbh);end  NameChangeFcn=if exist('rename_tlblock','file')==2,rename_tlblock(gcbh);end  OpenFcn=if exist('tl_open_blockdlg','file')==2,tl_open_blockdlg(gcbh);else,open_system(gcbh,'parameter');end
      mask Help: eval(['if exist(''tl_online_help'',''file'') == 2, tl_online_help(''Topic'',''TL_RelationalOperator''),else, web([''jar:file:///'',matlabroot,''/help/toolbox/simulink/help.jar!/slref/' lower(get_param(gcbh,'Blocktype')) '.html''], ''-helpbrowser''),end'])
      mask Display: plot([-0.05, 1.05, NaN, -0.05, 1.05],[.01, .01, NaN, .99, .99])
  Rescale Target : Constant  Value=ddv('BFE/ExecuteStdSteps_Rescaling/KU16_VOLT_RSC_NUM1')  mask(TL_Constant){data={'output',{'variable','BFE/ExecuteStdSteps_Rescaling/KU16_VOLT_RSC_NUM1'},'date',735951.66852160881}}
      settings: CopyFcn=if exist('tl_reset_reviewflag','file')==2,tl_reset_reviewflag(gcbh);end  DeleteFcn=if exist('delete_tlblock','file')==2,delete_tlblock(gcbh);end  NameChangeFcn=if exist('rename_tlblock','file')==2,rename_tlblock(gcbh);end  OpenFcn=if exist('tl_open_blockdlg','file')==2,tl_open_blockdlg(gcbh);else,open_system(gcbh,'parameter');end
      mask Help: eval(['if exist(''tl_online_help'',''file'') == 2, tl_online_help(''Topic'',''TL_Constant''),else, web([''jar:file:///'',matlabroot,''/help/toolbox/simulink/help.jar!/slref/' lower(get_param(gcbh,'Blocktype')) '.html''], ''-helpbrowser''),end'])
      mask Display: plot([-0.05, 1.05, NaN, -0.05, 1.05],[.01, .01, NaN, .99, .99])
  Sign : Signum  mask(TL_Signum){data={'output',{'name','s16TargetSign_$S'},'date',735951.66852094908}}
      settings: DeleteFcn=if exist('delete_tlblock','file')==2,delete_tlblock(gcbh);end  NameChangeFcn=if exist('rename_tlblock','file')==2,rename_tlblock(gcbh);end  OpenFcn=if exist('tl_open_blockdlg','file')==2,tl_open_blockdlg(gcbh);else,open_system(gcbh,'parameter');end
      mask Help: eval(['if exist(''tl_online_help'',''file'') == 2, tl_online_help(''Topic'',''TL_Signum''),else, web([''jar:file:///'',matlabroot,''/help/toolbox/simulink/help.jar!/slref/' lower(get_param(gcbh,'Blocktype')) '.html''], ''-helpbrowser''),end'])
      mask Display: plot([-0.05, 1.05, NaN, -0.05, 1.05],[.01, .01, NaN, .99, .99])
  Sum : Sum  mask(TL_Sum){data={'output',{'type','Int32'},'date',735951.66852067132}}
      settings: CopyFcn=if exist('tl_reset_reviewflag','file')==2,tl_reset_reviewflag(gcbh);end  DeleteFcn=if exist('delete_tlblock','file')==2,delete_tlblock(gcbh);end  NameChangeFcn=if exist('rename_tlblock','file')==2,rename_tlblock(gcbh);end  OpenFcn=if exist('tl_open_blockdlg','file')==2,tl_open_blockdlg(gcbh);else,open_system(gcbh,'parameter');end
      mask Help: eval(['if exist(''tl_online_help'',''file'') == 2, tl_online_help(''Topic'',''TL_Sum''),else, web([''jar:file:///'',matlabroot,''/help/toolbox/simulink/help.jar!/slref/' lower(get_param(gcbh,'Blocktype')) '.html''], ''-helpbrowser''),end'])
      mask Display: plot([-0.05, 1.05, NaN, -0.05, 1.05],[.01, .01, NaN, .99, .99])
  Switch : Switch  Criteria=u2 ~= 0  mask(TL_Switch){data={'output',{'name','u16BattVoltFiltered','type','UInt16'},'date',735951.66852027783}}
      settings: CopyFcn=if exist('tl_reset_reviewflag','file')==2,tl_reset_reviewflag(gcbh);end  DeleteFcn=if exist('delete_tlblock','file')==2,delete_tlblock(gcbh);end  NameChangeFcn=if exist('rename_tlblock','file')==2,rename_tlblock(gcbh);end  OpenFcn=if exist('tl_open_blockdlg','file')==2,tl_open_blockdlg(gcbh);else,open_system(gcbh,'parameter');end
      mask Help: eval(['if exist(''tl_online_help'',''file'') == 2, tl_online_help(''Topic'',''TL_Switch''),else, web([''jar:file:///'',matlabroot,''/help/toolbox/simulink/help.jar!/slref/' lower(get_param(gcbh,'Blocktype')) '.html''], ''-helpbrowser''),end'])
      mask Display: plot([-0.05, 1.05, NaN, -0.05, 1.05],[.01, .01, NaN, .99, .99])
  sUnsaturatedMotorPowerOrder : Outport
  wires:
  lOrderToApply/1 -> Sign/1, Product2/1
  Rescale Target/1 -> Product2/2
  Arrondi 1/2 lsb/1 -> Product/1
  Product1/1 -> Product4/1
  Protection for division by 0/1 -> Relational Operator/1
  Divider to rescale output/1 -> Product1/2
  Sum/1 -> Product1/1
  Product/1 -> Product3/2
  Relational Operator/1 -> Switch/2
  Switch/1 -> Product4/2
  usBatteryVoltage/1 -> Product3/1, Relational Operator/2, Switch/3
  Product4/1 -> sUnsaturatedMotorPowerOrder/1
  Product3/1 -> Sum/1
  Default value for Battery Voltage/1 -> Switch/1
  Product2/1 -> Sum/2
  Sign/1 -> Product/2

== system BFE_TestHarness/BFE_AC_BeltFunctionExecution/Subsystem/BFE_AC_BeltFunctionExecution/BFE_AC_BeltFunctionExecution/BFE_runExecuteStandardSteps/ExecuteStandardSteps/SubsystemConvertOrderToMotorPower/MotorVoltage_Regulation/Consign > Battery voltage => Saturate to MAX PWM ==
  lOrderToApply : Inport
  Action Port : ActionPort  ActionType=then
  Constant : Constant  Value=ddv('Common/KS32_ZERO')  mask(TL_Constant){data={'output',{'variable','Common/KS32_ZERO'},'date',737167.45535738429}}
      settings: CopyFcn=if exist('tl_reset_reviewflag') == 2, tl_reset_reviewflag(gcbh); end  DeleteFcn=if exist('delete_tlblock','file')==2,delete_tlblock(gcbh);end  NameChangeFcn=if exist('rename_tlblock','file')==2,rename_tlblock(gcbh);end  OpenFcn=if exist('tl_open_blockdlg','file')==2,tl_open_blockdlg(gcbh);else,open_system(gcbh,'parameter');end
      mask Help: eval(['if exist(''tl_online_help'',''file'') == 2, tl_online_help(''Topic'',''TL_Constant''),else, web([''jar:file:///'',matlabroot,''/help/toolbox/simulink/help.jar!/slref/' lower(get_param(gcbh,'Blocktype')) '.html''], ''-helpbrowser''),end'])
      mask Display: plot([-0.1, 1.05, NaN, -0.1, 1.05],[.01, .01, NaN, .99, .99]);
  Constant1 : Constant  Value=ddv('BFE/KS16_PWM_MAX_BTN')  mask(TL_Constant){data={'output',{'variable','BFE/KS16_PWM_MAX_BTN'},'date',737167.47128910874}}
      settings: CopyFcn=if exist('tl_reset_reviewflag') == 2, tl_reset_reviewflag(gcbh); end  DeleteFcn=if exist('delete_tlblock','file')==2,delete_tlblock(gcbh);end  NameChangeFcn=if exist('rename_tlblock','file')==2,rename_tlblock(gcbh);end  OpenFcn=if exist('tl_open_blockdlg','file')==2,tl_open_blockdlg(gcbh);else,open_system(gcbh,'parameter');end
      mask Help: eval(['if exist(''tl_online_help'',''file'') == 2, tl_online_help(''Topic'',''TL_Constant''),else, web([''jar:file:///'',matlabroot,''/help/toolbox/simulink/help.jar!/slref/' lower(get_param(gcbh,'Blocktype')) '.html''], ''-helpbrowser''),end'])
      mask Display: plot([-0.1, 1.05, NaN, -0.1, 1.05],[.01, .01, NaN, .99, .99]);
  Constant2 : Constant  Value=ddv('BFE/KS16_PWM_MIN_BTN')  mask(TL_Constant){data={'output',{'variable','BFE/KS16_PWM_MIN_BTN'},'date',737167.47139391198}}
      settings: CopyFcn=if exist('tl_reset_reviewflag') == 2, tl_reset_reviewflag(gcbh); end  DeleteFcn=if exist('delete_tlblock','file')==2,delete_tlblock(gcbh);end  NameChangeFcn=if exist('rename_tlblock','file')==2,rename_tlblock(gcbh);end  OpenFcn=if exist('tl_open_blockdlg','file')==2,tl_open_blockdlg(gcbh);else,open_system(gcbh,'parameter');end
      mask Help: eval(['if exist(''tl_online_help'',''file'') == 2, tl_online_help(''Topic'',''TL_Constant''),else, web([''jar:file:///'',matlabroot,''/help/toolbox/simulink/help.jar!/slref/' lower(get_param(gcbh,'Blocktype')) '.html''], ''-helpbrowser''),end'])
      mask Display: plot([-0.1, 1.05, NaN, -0.1, 1.05],[.01, .01, NaN, .99, .99]);
  Relational Operator : RelationalOperator  Operator=<  OutDataTypeStr=boolean  mask(TL_RelationalOperator){data={'date',737167.45277324074}}
      settings: DeleteFcn=if exist('delete_tlblock','file')==2,delete_tlblock(gcbh);end  NameChangeFcn=if exist('rename_tlblock','file')==2,rename_tlblock(gcbh);end  OpenFcn=if exist('tl_open_blockdlg','file')==2,tl_open_blockdlg(gcbh);else,open_system(gcbh,'parameter');end
      mask Help: eval(['if exist(''tl_online_help'',''file'') == 2, tl_online_help(''Topic'',''TL_RelationalOperator''),else, web([''jar:file:///'',matlabroot,''/help/toolbox/simulink/help.jar!/slref/' lower(get_param(gcbh,'Blocktype')) '.html''], ''-helpbrowser''),end'])
      mask Display: plot([-0.1, 1.05, NaN, -0.1, 1.05],[.01, .01, NaN, .99, .99]);
  SaturatedOrder : Switch  Criteria=u2 ~= 0  mask(TL_Switch){data={'output',{'type','Int32'},'date',737167.54835017363}}
      settings: CopyFcn=if exist('tl_reset_reviewflag') == 2, tl_reset_reviewflag(gcbh); end  DeleteFcn=if exist('delete_tlblock','file')==2,delete_tlblock(gcbh);end  NameChangeFcn=if exist('rename_tlblock','file')==2,rename_tlblock(gcbh);end  OpenFcn=if exist('tl_open_blockdlg','file')==2,tl_open_blockdlg(gcbh);else,open_system(gcbh,'parameter');end
      mask Help: eval(['if exist(''tl_online_help'',''file'') == 2, tl_online_help(''Topic'',''TL_Switch''),else, web([''jar:file:///'',matlabroot,''/help/toolbox/simulink/help.jar!/slref/' lower(get_param(gcbh,'Blocktype')) '.html''], ''-helpbrowser''),end'])
      mask Display: plot([-0.1, 1.05, NaN, -0.1, 1.05],[.01, .01, NaN, .99, .99]);
  sUnsaturatedMotorPowerOrder : Outport
  wires:
  lOrderToApply/1 -> Relational Operator/1
  Constant/1 -> Relational Operator/2
  Relational Operator/1 -> SaturatedOrder/2
  Constant2/1 -> SaturatedOrder/1
  Constant1/1 -> SaturatedOrder/3
  SaturatedOrder/1 -> sUnsaturatedMotorPowerOrder/1

== system BFE_TestHarness/BFE_AC_BeltFunctionExecution/Subsystem/BFE_AC_BeltFunctionExecution/BFE_AC_BeltFunctionExecution/BFE_runExecuteStandardSteps/ExecuteStandardSteps/SubsystemConvertOrderToMotorPower/RescaleOrderType/If Action Subsystem ==
  In1 : Inport
  Action Port : ActionPort  ActionType=then
  8Bit Decoder : Subsystem  RequirementInfo={} %GIDa_46c16828_8e89_4125_87c7_825d83414c22  mask(TLSAMPLES_8BIT_DECODER){}
      mask help:
      | Decodes one UInt8 byte into 8 bits.
      | All inputs are boolean variables.
      |
      | Sample implementation using TargetLink Custom Code block.
      | Version 1.0.
  Gain : Gain  RequirementInfo={} %GIDa_463ccd80_c379_4bfe_b2d9_3dc830b3b5e8  Gain=2  mask(TL_Gain){data={'output',{'type','UInt8'},'date',735951.66851472226}}
      settings: CopyFcn=if exist('tl_reset_reviewflag','file')==2,tl_reset_reviewflag(gcbh);end  DeleteFcn=if exist('delete_tlblock','file')==2,delete_tlblock(gcbh);end  NameChangeFcn=if exist('rename_tlblock','file')==2,rename_tlblock(gcbh);end  OpenFcn=if exist('tl_open_blockdlg','file')==2,tl_open_blockdlg(gcbh);else,open_system(gcbh,'parameter');end
      mask Help: eval(['if exist(''tl_online_help'',''file'') == 2, tl_online_help(''Topic'',''TL_Gain''),else, web([''jar:file:///'',matlabroot,''/help/toolbox/simulink/help.jar!/slref/' lower(get_param(gcbh,'Blocktype')) '.html''], ''-helpbrowser''),end'])
      mask Display: plot([0, .9, 0],[.05, .5, .95])
  Gain1 : Gain  RequirementInfo={} %GIDa_53a4e368_9e8e_4733_ab15_169b38b41554  Gain=4  mask(TL_Gain){data={'output',{'type','UInt8'},'date',735951.66851418978}}
      settings: CopyFcn=if exist('tl_reset_reviewflag','file')==2,tl_reset_reviewflag(gcbh);end  DeleteFcn=if exist('delete_tlblock','file')==2,delete_tlblock(gcbh);end  NameChangeFcn=if exist('rename_tlblock','file')==2,rename_tlblock(gcbh);end  OpenFcn=if exist('tl_open_blockdlg','file')==2,tl_open_blockdlg(gcbh);else,open_system(gcbh,'parameter');end
      mask Help: eval(['if exist(''tl_online_help'',''file'') == 2, tl_online_help(''Topic'',''TL_Gain''),else, web([''jar:file:///'',matlabroot,''/help/toolbox/simulink/help.jar!/slref/' lower(get_param(gcbh,'Blocktype')) '.html''], ''-helpbrowser''),end'])
      mask Display: plot([0, .9, 0],[.05, .5, .95])
  Rescaler : DataTypeConversion  RequirementInfo={} %GIDa_460a69a1_ea43_46e4_beee_dc01686cf286  OutDataTypeStr=boolean  SaturateOnIntegerOverflow=on  RndMeth=Zero  mask(TL_Rescaler){data={'output',{'type','Bool'},'date',735951.6685136921}}
      settings: DeleteFcn=if exist('delete_tlblock','file')==2,delete_tlblock(gcbh);end  NameChangeFcn=if exist('rename_tlblock','file')==2,rename_tlblock(gcbh);end  OpenFcn=if exist('tl_open_blockdlg','file')==2,tl_open_blockdlg(gcbh);else,open_system(gcbh,'parameter');end
      mask Help: eval(['if exist(''tl_online_help'',''file'') == 2, tl_online_help(''Topic'',''TL_Rescaler''),else, web([''jar:file:///'',matlabroot,''/help/toolbox/simulink/help.jar!/slref/' lower(get_param(gcbh,'Blocktype')) '.html''], ''-helpbrowser''),end'])
      mask Display: plot([-0.05, 1.05, NaN, -0.05, 1.05],[.01, .01, NaN, .99, .99])
  Rescaler1 : DataTypeConversion  RequirementInfo={} %GIDa_2f15a786_e57c_4995_997a_da46f3f20525  OutDataTypeStr=boolean  SaturateOnIntegerOverflow=on  RndMeth=Zero  mask(TL_Rescaler){data={'output',{'type','Bool'},'date',735951.66851335648}}
      settings: DeleteFcn=if exist('delete_tlblock','file')==2,delete_tlblock(gcbh);end  NameChangeFcn=if exist('rename_tlblock','file')==2,rename_tlblock(gcbh);end  OpenFcn=if exist('tl_open_blockdlg','file')==2,tl_open_blockdlg(gcbh);else,open_system(gcbh,'parameter');end
      mask Help: eval(['if exist(''tl_online_help'',''file'') == 2, tl_online_help(''Topic'',''TL_Rescaler''),else, web([''jar:file:///'',matlabroot,''/help/toolbox/simulink/help.jar!/slref/' lower(get_param(gcbh,'Blocktype')) '.html''], ''-helpbrowser''),end'])
      mask Display: plot([-0.05, 1.05, NaN, -0.05, 1.05],[.01, .01, NaN, .99, .99])
  Sum : Sum  RequirementInfo={} %GIDa_7349fd7c_8e3a_490a_b493_eadf84edf145  Inputs=+++  OutDataTypeStr=uint8  mask(TL_Sum){data={'output',{'type','UInt8'},'date',735951.66851304402}}
      settings: CopyFcn=if exist('tl_reset_reviewflag','file')==2,tl_reset_reviewflag(gcbh);end  DeleteFcn=if exist('delete_tlblock','file')==2,delete_tlblock(gcbh);end  NameChangeFcn=if exist('rename_tlblock','file')==2,rename_tlblock(gcbh);end  OpenFcn=if exist('tl_open_blockdlg','file')==2,tl_open_blockdlg(gcbh);else,open_system(gcbh,'parameter');end
      mask Help: eval(['if exist(''tl_online_help'',''file'') == 2, tl_online_help(''Topic'',''TL_Sum''),else, web([''jar:file:///'',matlabroot,''/help/toolbox/simulink/help.jar!/slref/' lower(get_param(gcbh,'Blocktype')) '.html''], ''-helpbrowser''),end'])
      mask Display: plot([-0.05, 1.05, NaN, -0.05, 1.05],[.01, .01, NaN, .99, .99])
  Terminator : Terminator
      settings: RequirementInfo={} %GIDa_034f8cba_dfaf_4414_8c6b_6ab8080e4773
  Terminator1 : Terminator
      settings: RequirementInfo={} %GIDa_499b6c5f_c858_4295_a2f0_b95703c00fe4
  Terminator2 : Terminator
      settings: RequirementInfo={} %GIDa_95669027_5da4_48d2_a1a6_bee5f704bf2b
  OrderType_Rescaled : Outport  RequirementInfo={} %GIDa_05e1c97c_70b1_4c9d_8ebf_6d017c5a3f14  InitialOutput=7
  bIsPID_M : Outport  RequirementInfo={} %GIDa_b0c3c1c0_9bc5_4551_96ea_6be82bcb0510  Port=2  InitialOutput=0
  IsPID_S : Outport  RequirementInfo={} %GIDa_e6a3f575_7609_4229_a4ea_de6723c8ce5e  Port=3  InitialOutput=0
  wires:
  In1/1 -> 8Bit Decoder/1(U8in)
  8Bit Decoder/4(Bit4) -> Rescaler1/1
  8Bit Decoder/3(Bit5) -> Rescaler/1
  8Bit Decoder/1(Bit7) -> Terminator/1
  8Bit Decoder/2(Bit6) -> Terminator1/1
  Rescaler/1 -> bIsPID_M/1
  Rescaler1/1 -> IsPID_S/1
  8Bit Decoder/5(Bit3) -> Terminator2/1
  8Bit Decoder/6(Bit2) -> Gain1/1
  8Bit Decoder/7(Bit1) -> Gain/1
  Gain1/1 -> Sum/1
  Gain/1 -> Sum/2
  8Bit Decoder/8(Bit0) -> Sum/3
  Sum/1 -> OrderType_Rescaled/1
